simulink model "q_ball_beam_control"  (R2019a)
settings: Solver=ode4  StartTime=0.0  StopTime=inf  FixedStep=0.002  RelTol=1e-3
values from neighbouring files (symbols this model uses):
  Kc = 5.3    [setup_ball_beam.m]    (also in setup_ball_beam_OG.m = 0.5)
  wf = 2 * pi * 4.0    (= 25.1327412287)    [setup_ball_beam.m]    (also in setup_ball_beam_OG.m)
  z = 1.4    [setup_ball_beam.m]    (also in setup_ball_beam_OG.m = 1)
undefined symbols (not defined in the file or in its folder): HIL, qc_get_step_size
libraries: quarc_library x4, simulink_extras x2
settings Model: ExtModeTrigDuration=12500  Creator=MLevis  LastModifiedBy=pmartin
settings DataIOCC: ReturnWorkspaceOutputs=off
settings DebuggingCC: UnderspecifiedInitializationDetection=Classic  MergeDetectMultiDrivingBlocksExec=none
settings ModelReferenceCC: PropagateSignalLabelsOutOfModel=off

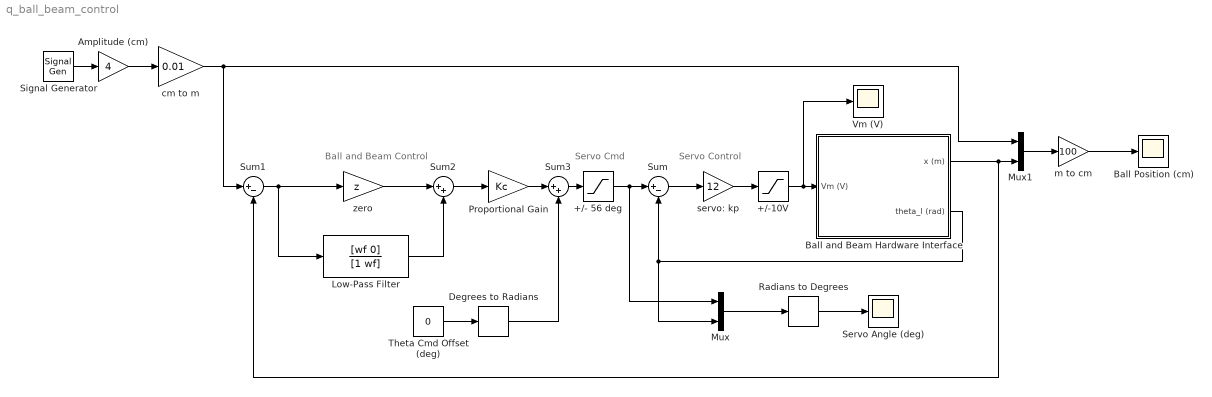
== system q_ball_beam_control ==
  note: Servo Cmd
  note: Servo Control
  note: Ball and Beam Control
  +/- 56 deg : Saturate  UpperLimit=56*pi/180  LowerLimit=-56*pi/180
  +/-10V : Saturate  UpperLimit=10  LowerLimit=-10
  Amplitude (cm) : Gain  Gain=4
  Ball Position (cm) : Scope
  Ball and Beam Hardware Interface : Subsystem
  Degrees to Radians : simulink_extras/Transformations/Degrees to Radians
  Low-Pass Filter : TransferFcn  Numerator=[wf 0]  Denominator=[1 wf]
  Mux : Mux  Inputs=2
  Mux1 : Mux  Inputs=2
  Proportional Gain : Gain  Gain=Kc
  Radians to Degrees : simulink_extras/Transformations/Radians to Degrees
  Servo Angle (deg) : Scope
  Signal Generator : SignalGenerator  WaveForm=square  Frequency=0.075
  Sum : Sum  Inputs=|+-
  Sum1 : Sum  Inputs=|+-
  Sum2 : Sum  Inputs=|++
  Sum3 : Sum  Inputs=|++
  Theta Cmd Offset (deg) : Constant  Value=0
  Vm (V) : Scope
  cm to m : Gain  Gain=0.01
  m to cm : Gain  Gain=100
  servo: kp : Gain  Gain=12
  zero : Gain  Gain=z
  wires:
  Radians to Degrees/1 -> Servo Angle (deg)/1
  Mux/1 -> Radians to Degrees/1
  Mux1/1 -> m to cm/1
  m to cm/1 -> Ball Position (cm)/1
  Amplitude (cm)/1 -> cm to m/1
  cm to m/1 -> Sum1/1, Mux1/1
  Sum/1 -> servo: kp/1
  Signal Generator/1 -> Amplitude (cm)/1
  servo: kp/1 -> +/-10V/1
  +/- 56 deg/1 -> Sum/1, Mux/1
  Ball and Beam Hardware Interface/2(theta_l (rad)) -> Sum/2, Mux/2
  Ball and Beam Hardware Interface/1(x (m)) -> Mux1/2, Sum1/2
  zero/1 -> Sum2/1
  Sum2/1 -> Proportional Gain/1
  Low-Pass Filter/1 -> Sum2/2
  Sum1/1 -> Low-Pass Filter/1, zero/1
  +/-10V/1 -> Vm (V)/1, Ball and Beam Hardware Interface/1(Vm (V))
  Sum3/1 -> +/- 56 deg/1
  Theta Cmd Offset (deg)/1 -> Degrees to Radians/1
  Proportional Gain/1 -> Sum3/1
  Degrees to Radians/1 -> Sum3/2

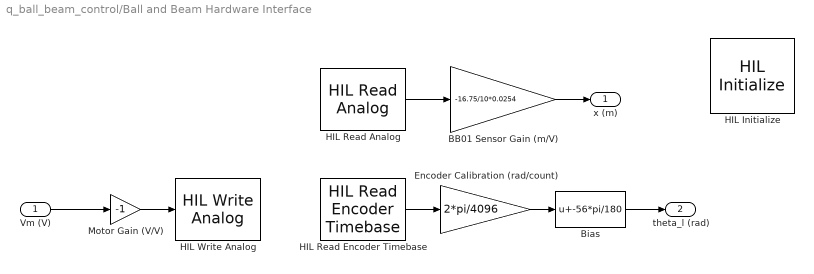
== system q_ball_beam_control/Ball and Beam Hardware Interface ==
  Vm (V) : Inport
  BB01 Sensor Gain (m/V) : Gain  Gain=-16.75/10*0.0254
  Bias : Bias  Bias=-56*pi/180
  Encoder Calibration (rad/count) : Gain  Gain=2*pi/4096  SaturateOnIntegerOverflow=on  OutDataTypeStr=Inherit: Same as input  ParamDataTypeStr=Inherit: Same as input
  HIL Initialize : quarc_library/Data Acquisition/Generic/Configuration/HIL Initialize  object_name=HIL-1  board_type=q8_usb  board_number=0@tcpip://localhost:18942  board_options=update_rate=normal  exclusive=off  active=on  hardware_clocks=[0:2]  clock_modes=[]  initial_clock_frequencies=[]  set_clock_params_at_start=off  set_clock_params_at_switch_in=off  set_clock_frequencies_at_start=off  set_clock_frequencies_at_switch_in=off  analog_input_channels=[0:7]  analog_input_configurations=[]  analog_input_maximums=10  analog_input_minimums=-10  set_analog_input_params_at_start=on  set_analog_input_params_at_switch_in=off  analog_output_channels=[0:7]  analog_output_maximums=10  analog_output_minimums=-10  initial_analog_outputs=[0]  final_analog_outputs=[0]  watchdog_analog_outputs=0  set_analog_output_params_at_start=on  set_analog_output_params_at_switch_in=off  set_analog_outputs_at_start=on  set_analog_outputs_at_switch_in=off  set_analog_outputs_at_terminate=on  set_analog_outputs_at_switch_out=off  set_analog_outputs_on_watchdog=off  digital_input_channels=[]  digital_output_channels=[0:7]  digital_output_configuration=[]  initial_digital_outputs=[0]  final_digital_outputs=[0]  watchdog_digital_outputs=[0]  set_digital_output_params_at_start=off  set_digital_output_params_at_switch_in=off  set_digital_outputs_at_start=on  set_digital_outputs_at_switch_in=off  set_digital_outputs_at_terminate=on  set_digital_outputs_at_switch_out=off  set_digital_outputs_on_watchdog=off  encoder_channels=[0:7]  quadrature=[4]  encoder_filter_frequency=[]  initial_encoder_counts=[0]  set_encoder_params_at_start=on  set_encoder_params_at_switch_in=off  set_encoder_counts_at_start=on  set_encoder_counts_at_switch_in=off  pwm_channels=[0:7]  pwm_modes=0  pwm_frequency=99.532799999999995e6/4095  pwm_configuration=[0]  pwm_alignment=[0]  pwm_polarity=[1]  pwm_leading_deadband=[0]  pwm_trailing_deadband=[0]  initial_pwm_outputs=[0]  final_pwm_outputs=[0]  watchdog_pwm_outputs=[0]  set_pwm_params_at_start=on  set_pwm_params_at_switch_in=off  set_pwm_outputs_at_start=on  set_pwm_outputs_at_switch_in=off  set_pwm_outputs_at_terminate=on  set_pwm_outputs_at_switch_out=off  set_pwm_outputs_on_watchdog=off  other_output_channels=[]  initial_other_outputs=[]  final_other_outputs=[]  watchdog_other_outputs=[]  set_other_outputs_at_start=off  set_other_outputs_at_switch_in=off  set_other_outputs_at_terminate=off  set_other_outputs_at_switch_out=off  set_other_outputs_on_watchdog=off
  HIL Read Analog : quarc_library/Data Acquisition/Generic/Immediate I//O/HIL Read Analog  object_name=HIL-1  channels=[0]  sample_time=qc_get_step_size  active=on  vector_output=off
  HIL Read Encoder Timebase : quarc_library/Data Acquisition/Generic/Timebases/HIL Read Encoder Timebase  object_name=HIL-1  clock=0  channels=0  active=on  vector_output=off  data_type_mode=Inherit via back propagation  data_type=double  overflow_mode=Synchronize (for simulated cards only)  samples_in_buffer=1 + 0 * max(ceil(1/qc_get_step_size), 1)
  HIL Write Analog : quarc_library/Data Acquisition/Generic/Immediate I//O/HIL Write Analog  Tag=unassigned  object_name=HIL-1  channels=0  sample_time=-1  active=on  vector_input=off
  Motor Gain (V/V) : Gain  Gain=-1
  x (m) : Outport
  theta_l (rad) : Outport  Port=2
  wires:
  HIL Read Encoder Timebase/1 -> Encoder Calibration (rad/count)/1
  Encoder Calibration (rad/count)/1 -> Bias/1
  HIL Read Analog/1 -> BB01 Sensor Gain (m/V)/1
  Vm (V)/1 -> Motor Gain (V/V)/1
  Motor Gain (V/V)/1 -> HIL Write Analog/1
  Bias/1 -> theta_l (rad)/1
  BB01 Sensor Gain (m/V)/1 -> x (m)/1
